simulink model "simulationjake"  (R2019a)
settings: Solver=VariableStepAuto  StartTime=0.0  StopTime=10.0  RelTol=1e-3
undefined symbols (not defined in the file or in its folder): u0, uin
libraries: simulink x1
settings Model: Creator=hyeokjae  LastModifiedBy=hyeokjae

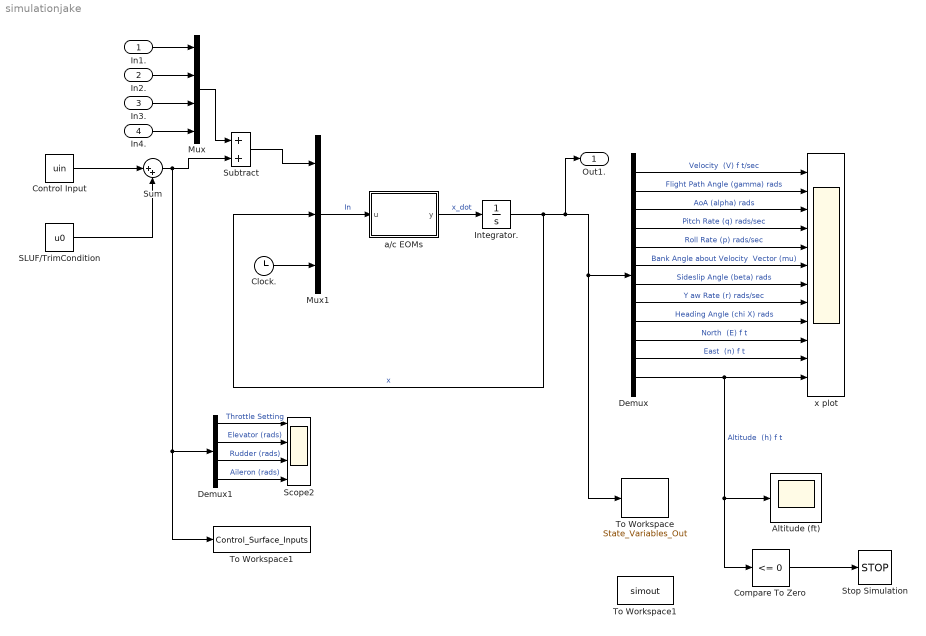
== system simulationjake ==
  In1. : Inport
  In2. : Inport  Port=2
  In3. : Inport  Port=3
  In4. : Inport  Port=4
  Altitude (ft) : Scope
  Clock. : Clock
  "Compare To Zero " : simulink/Logic and Bit Operations/Compare To Zero  relop=<=  OutDataTypeStr=boolean
  Control Input : Constant  Value=uin
  Demux : Demux  Outputs=12
  Demux1 : Demux
  Integrator. : Integrator
  Mux : Mux
  Mux1 : Mux  Inputs=3
  "SLUF/TrimCondition " : Constant  Value=u0
  Scope2 : Scope  NumInputPorts=4
  "Stop Simulation " : Stop
  Subtract : Sum
  Sum : Sum  Inputs=|++
  "To Workspace " : ToWorkspace  VariableName=State_Variables_Out  SampleTime=-1
      settings: Save2DSignal=2-D array (concatenate along first dimension)
  To Workspace1 : ToWorkspace  VariableName=simout  SaveFormat=Timeseries  SampleTime=-1
  "To Workspace1 " : ToWorkspace  VariableName=Control_Surface_Inputs  SampleTime=-1
      settings: Save2DSignal=2-D array (concatenate along first dimension)
  a/c EOMs : MATLAB Function  TreatAsAtomicUnit=on
  x plot : Scope  NumInputPorts=12
  Out1. : Outport
  wires:
  Control Input/1 -> Sum/1
  "SLUF/TrimCondition "/1 -> Sum/2
  In4./1 -> Mux/4
  In3./1 -> Mux/3
  In2./1 -> Mux/2
  In1./1 -> Mux/1
  Sum/1 -> "To Workspace1 "/1, Demux1/1, Subtract/2
  Mux/1 -> Subtract/1
  Subtract/1 -> Mux1/1
  Mux1/1 -> a/c EOMs/1(u)  "In"
  a/c EOMs/1(y) -> Integrator./1  "x_dot"
  Integrator./1 -> Mux1/2, Out1./1, "To Workspace "/1, Demux/1  "x"
  Demux/1 -> x plot/1  "Velocity  (V) f t/sec"
  Demux/2 -> x plot/2  "Flight Path Angle (gamma) rads"
  Demux/3 -> x plot/3  "AoA (alpha) rads"
  Demux/4 -> x plot/4  "Pitch Rate (q) rads/sec"
  Demux/5 -> x plot/5  "Roll Rate (p) rads/sec"
  Demux/6 -> x plot/6  "Bank Angle about Velocity  Vector (mu)"
  Demux/7 -> x plot/7  "Sideslip Angle (beta) rads"
  Demux/8 -> x plot/8  "Y aw Rate (r) rads/sec"
  Demux/9 -> x plot/9  "Heading Angle (chi X) rads"
  Demux/10 -> x plot/10  "North  (E) f t"
  Demux/11 -> x plot/11  "East  (n) f t"
  Demux/12 -> "Compare To Zero "/1, Altitude (ft)/1, x plot/12  "Altitude  (h) f t"
  Clock./1 -> Mux1/3
  "Compare To Zero "/1 -> "Stop Simulation "/1
  Demux1/1 -> Scope2/1  "Throttle Setting"
  Demux1/2 -> Scope2/2  "Elevator (rads)"
  Demux1/3 -> Scope2/3  "Rudder (rads)"
  Demux1/4 -> Scope2/4  "Aileron (rads)"

== matlab function simulationjake/a//c EOMs ==
  data: u input; y output
function y = fcn(u)

y = u;
